simulink model "model_prob_4"  (R2016a)
settings: Solver=FixedStepDiscrete  StartTime=0.0  StopTime=10.0  RelTol=1e-3
values from neighbouring files (symbols this model uses):
  a0 = 0.25    [MAT-file_prob_4.mat]
  a1 = 0.5    [MAT-file_prob_4.mat]
  a2 = 0.4    [MAT-file_prob_4.mat]
libraries: simulink x1
settings Model: Creator=Admin  LastModifiedBy=Admin
settings DataIOCC: ExternalInput=[t, in]  LoadExternalInput=on

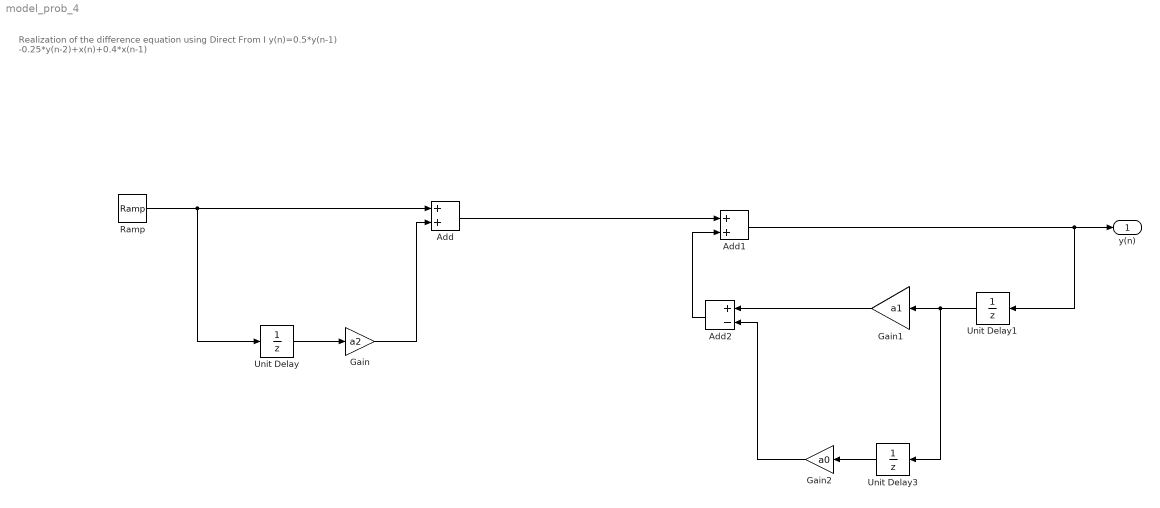
== system model_prob_4 ==
  note: Realization of the difference equation using Direct From I
      |
      | y(n)=0.5*y(n-1) -0.25*y(n-2)+x(n)+0.4*x(n-1)
  Add : Sum
  Add1 : Sum
  Add2 : Sum  Inputs=+-
  Gain : Gain  Gain=a2
  Gain1 : Gain  Gain=a1
  Gain2 : Gain  Gain=a0
  Ramp : simulink/Sources/Ramp  slope=1  start=0  X0=0
  Unit Delay : UnitDelay  SampleTime=-1
  Unit Delay1 : UnitDelay  SampleTime=-1
  Unit Delay3 : UnitDelay  SampleTime=-1
  y(n) : Outport
  wires:
  Ramp/1 -> Unit Delay/1, Add/1
  Unit Delay/1 -> Gain/1
  Gain/1 -> Add/2
  Add/1 -> Add1/1
  Add1/1 -> Unit Delay1/1, y(n)/1
  Add2/1 -> Add1/2
  Unit Delay1/1 -> Unit Delay3/1, Gain1/1
  Gain1/1 -> Add2/1
  Unit Delay3/1 -> Gain2/1
  Gain2/1 -> Add2/2
